simulink model "modelo_q1"  (R2016a)
settings: Solver=VariableStepAuto  StartTime=0.0  StopTime=20  MaxStep=0.001  RelTol=1e-3
values from neighbouring files (symbols this model uses):
  A = [(sin(th1)-sin(th1+2*th2))/(-3+cos(2*th2))  , (-sin(th1)+3*sin(th1+th2)-sin(th1-th2)+sin(th1+2*th2))/(-3+cos(2*th2)) ... (first row only)    [ajuda.m]    (also in controledesacoplante.m; gazebo_parameters.m = Amd; geracao.m = 0; gpc.m = [1.0013 0 0.0050)
  B = Bmd    [gazebo_parameters.m]    (also in geracao.m = 1; gpc.m = [-0.001; kalman_filter.m; questao1.m = double(subs(u, [x1 x2],[0 0])))
  C = Cm    [gazebo_parameters.m]    (also in geracao.m = -1; gpc.m = [1 0 0; kalman_filter.m; questao1.m = [1 0 0)
  D = 0    [geracao.m]    (also in gpc.m = zeros(3,1); questao1.m = zeros(3,1))
  Ka = lqr(A, B, Q, R)    [questao1.m]
  L = Lkf    [questao1.m]
  Lkf = dlqr(Amd',Cm',1e-4*eye(3),1*eye(2))'    [gazebo_parameters.m]    (also in kalman_filter.m; questao1.m = Lkf')
  V1 = 0.0001*eye(3)    [questao1.m]
  V2 = 0.000005*eye(2)    [questao1.m]
  x0 = [pi/180*30 0 0]    [questao1.m]
  x0obs = [pi/180*45 ; 0; 0]    [questao1.m]
undefined symbols (not defined in the file or in its folder): sigbuilder_block
libraries: simulink x5
settings Model: Creator=Regner  LastModifiedBy=Regner

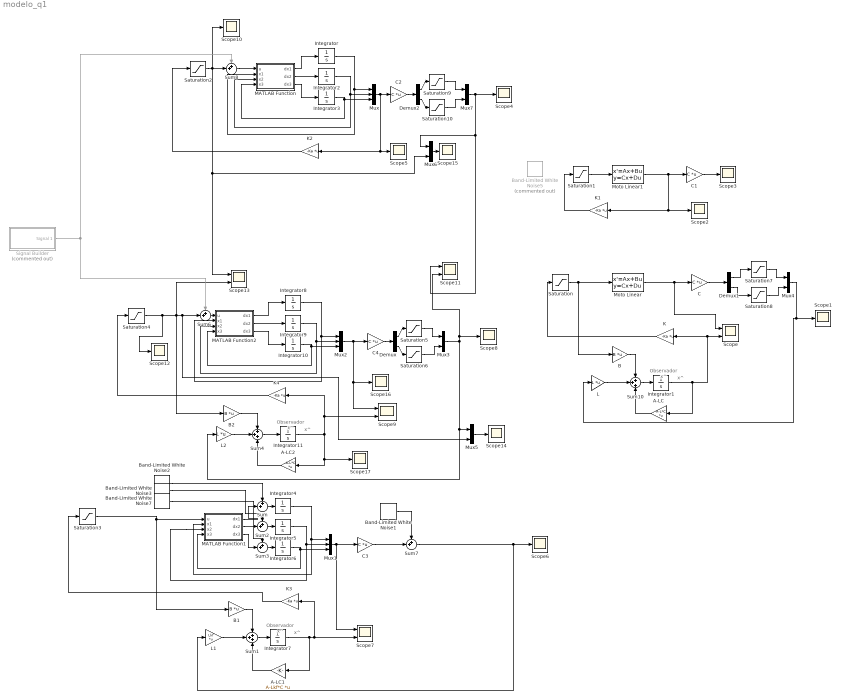
== system modelo_q1 ==
  note: Observador
  note: x^
  note: x^
  note: Observador
  note: x^
  note: x^
  note: Observador
  note: x^
  note: x^
  A-LC : Gain  Gain=A-L*C  Multiplication=Matrix(K*u)
  A-LC1 : Gain  Gain=A-Lkf*C  Multiplication=Matrix(K*u)
  A-LC2 : Gain  Gain=A-L*C  Multiplication=Matrix(K*u)
  B : Gain  Gain=B  Multiplication=Matrix(K*u)
  B1 : Gain  Gain=B  Multiplication=Matrix(K*u)
  B2 : Gain  Gain=B  Multiplication=Matrix(K*u)
  Band-Limited White Noise1 : simulink/Sources/Band-Limited White Noise  Cov=diag(V2)  Ts=0.1  seed=[23341]
  Band-Limited White Noise2 : simulink/Sources/Band-Limited White Noise  Cov=V1(1,1)  Ts=0.1  seed=[23341]
  Band-Limited White Noise3 : simulink/Sources/Band-Limited White Noise  Cov=V1(2,2)  Ts=0.1  seed=[23341]
  Band-Limited White Noise5 : simulink/Sources/Band-Limited White Noise  Commented=on  Cov=diag(V1)  Ts=0.1  seed=[23341]
  Band-Limited White Noise7 : simulink/Sources/Band-Limited White Noise  Cov=V1(3,3)  Ts=0.1  seed=[23341]
  C{,1..4} (5 alike) : Gain  Gain=C  Multiplication=Matrix(K*u)
  Demux : Demux  Outputs=2
  Demux1 : Demux  Outputs=2
  Demux2 : Demux  Outputs=2
  Integrator : Integrator  InitialCondition=x0(1)
  Integrator1 : Integrator  InitialCondition=x0obs
  Integrator10 : Integrator  InitialCondition=x0(3)
  Integrator11 : Integrator  InitialCondition=x0obs
  Integrator2 : Integrator  InitialCondition=x0(2)
  Integrator3 : Integrator  InitialCondition=x0(3)
  Integrator4 : Integrator  InitialCondition=x0(1)
  Integrator5 : Integrator  InitialCondition=x0(2)
  Integrator6 : Integrator  InitialCondition=x0(3)
  Integrator7 : Integrator  InitialCondition=x0obs
  Integrator8 : Integrator  InitialCondition=x0(1)
  Integrator9 : Integrator  InitialCondition=x0(2)
  K{,1..4} (5 alike) : Gain  Gain=-Ka  Multiplication=Matrix(K*u)
  L : Gain  Gain=L  Multiplication=Matrix(K*u)
  L1 : Gain  Gain=Lkf  Multiplication=Matrix(K*u)
  L2 : Gain  Gain=L  Multiplication=Matrix(K*u)
  MATLAB Function : MATLAB Function  TreatAsAtomicUnit=on
  MATLAB Function1 : MATLAB Function  TreatAsAtomicUnit=on
  MATLAB Function2 : MATLAB Function  TreatAsAtomicUnit=on
  Moto Linear : StateSpace  A=A  B=B  C=eye(3)  D=D  X0=x0
  Moto Linear1 : StateSpace  A=A  B=B  C=eye(3)  D=D  X0=x0
  Mux : Mux  Inputs=3
  Mux1 : Mux  Inputs=3
  Mux2 : Mux  Inputs=3
  Mux{3..7} (5 alike) : Mux  Inputs=2
  Saturation : Saturate  UpperLimit=50  LowerLimit=-50  ZeroCross=off
  Saturation1 : Saturate  UpperLimit=100  LowerLimit=-100  ZeroCross=off
  Saturation{5..6,9..10} (4 alike) : Saturate  UpperLimit=pi/4  LowerLimit=-pi/4
  Saturation2 : Saturate  UpperLimit=pi/2  LowerLimit=-pi/2  ZeroCross=off
  Saturation3 : Saturate  UpperLimit=inf  LowerLimit=-inf  ZeroCross=off
  Saturation4 : Saturate  UpperLimit=100  LowerLimit=-100  ZeroCross=off
  Saturation7 : Saturate  UpperLimit=pi  LowerLimit=-pi
  Saturation8 : Saturate  UpperLimit=pi  LowerLimit=-pi
  Scope{,7,9,11,13} (5 alike) : Scope  NumInputPorts=2
  Scope{1..6,8,10,12,14..17} (13 alike) : Scope
  Signal Builder : Subsystem  Tag=STV Subsys  Commented=on  LoadFcn=sigbuilder_block('load');  StartFcn=sigbuilder_block('start');  StopFcn=sigbuilder_block('stop');  ClipboardFcn=sigbuilder_block('clipboard');  mask(Sigbuilder block){}
      mask help: Simulink:masks:SigbuilderBlock_MD
      mask init:
      | if ~strcmp(get_param(bdroot(gcbh),'SimulationStatus'),'stopped') tuvar = sigbuilder_block('maskInit'); end
      settings: CopyFcn=sigbuilder_block('copy');  DeleteFcn=sigbuilder_block('delete');  ModelCloseFcn=sigbuilder_block('modelClose');  PreSaveFcn=sigbuilder_block('preSave');  PauseFcn=sigbuilder_block('pause');  ContinueFcn=sigbuilder_block('continue');  NameChangeFcn=sigbuilder_block('namechange');  OpenFcn=sigbuilder_block('open',[437.6 199.2 550.4 400 ]);  CloseFcn=sigbuilder_block('close');
      mask Display: plot(0, 0, 100, 100,[2, 2, 32, 32, 2], [68, 8, 8, 68, 68],[32, 2], [38, 38], [32, 19, 2],[53, 60, 44], [32, 17, 17, 2],[16, 16, 31, 31]);txt = getActiveGroup(gcbh);text(2, 100, txt,'verticalAlignment', 'top');
  Sum{,2..3,6..8} (6 alike) : Sum  Inputs=++|
  Sum1 : Sum  Inputs=+++
  Sum10 : Sum  Inputs=+++
  Sum4 : Sum  Inputs=+++
  wires:
  Moto Linear/1 -> C/1, Scope/1
  K/1 -> Saturation/1
  Mux4/1 -> L/1, Scope1/1
  Saturation1/1 -> Moto Linear1/1
  Moto Linear1/1 -> C1/1, Scope2/1, K1/1
  K1/1 -> Saturation1/1
  C1/1 -> Scope3/1
  Sum10/1 -> Integrator1/1
  L/1 -> Sum10/2
  A-LC/1 -> Sum10/3
  Integrator1/1 -> A-LC/1, Scope/2, K/1
  B/1 -> Sum10/1
  MATLAB Function/1(dx1) -> Integrator/1
  MATLAB Function/2(dx2) -> Integrator2/1
  MATLAB Function/3(dx3) -> Integrator3/1
  Integrator3/1 -> Mux/3, MATLAB Function/4(x3)
  Integrator2/1 -> Mux/2, MATLAB Function/3(x2)
  Integrator/1 -> Mux/1, MATLAB Function/2(x1)
  Saturation2/1 -> Sum8/2, Mux6/2, Scope13/1, Scope10/1
  Mux/1 -> Scope5/1, K2/1, C2/1
  K2/1 -> Saturation2/1
  MATLAB Function1/1(dx1) -> Sum/2
  MATLAB Function1/2(dx2) -> Sum2/2
  MATLAB Function1/3(dx3) -> Sum3/2
  K3/1 -> Saturation3/1
  Sum7/1 -> L1/1, Scope6/1
  Mux1/1 -> Scope7/1, C3/1
  Sum1/1 -> Integrator7/1
  L1/1 -> Sum1/2
  A-LC1/1 -> Sum1/3
  Integrator7/1 -> K3/1, Scope7/2, A-LC1/1
  B1/1 -> Sum1/1
  Band-Limited White Noise1/1 -> Sum7/1
  Saturation3/1 -> MATLAB Function1/1(u), B1/1
  MATLAB Function2/1(dx1) -> Integrator8/1
  MATLAB Function2/2(dx2) -> Integrator9/1
  MATLAB Function2/3(dx3) -> Integrator10/1
  Integrator10/1 -> Mux2/3, MATLAB Function2/4(x3)
  Integrator9/1 -> Mux2/2, MATLAB Function2/3(x2)
  Integrator8/1 -> Mux2/1, MATLAB Function2/2(x1)
  K4/1 -> Saturation4/1
  Mux3/1 -> Mux5/1, L2/1, Scope11/2, Scope8/1
  Saturation4/1 -> Scope12/1, Mux5/2, Sum6/2, Scope13/2, B2/1
  Mux2/1 -> C4/1, Scope16/1, Scope9/1
  Sum4/1 -> Integrator11/1
  L2/1 -> Sum4/2
  A-LC2/1 -> Sum4/3
  Integrator11/1 -> K4/1, Scope9/2, Scope17/1, A-LC2/1
  B2/1 -> Sum4/1
  Saturation/1 -> B/1, Moto Linear/1
  Integrator4/1 -> MATLAB Function1/2(x1), Mux1/1
  Integrator5/1 -> MATLAB Function1/3(x2), Mux1/2
  Integrator6/1 -> MATLAB Function1/4(x3), Mux1/3
  Band-Limited White Noise7/1 -> Sum3/1
  Band-Limited White Noise3/1 -> Sum2/1
  Band-Limited White Noise2/1 -> Sum/1
  C3/1 -> Sum7/2
  Mux7/1 -> Scope11/1, Mux6/1, Scope4/1
  Sum6/1 -> MATLAB Function2/1(u)
  Sum8/1 -> MATLAB Function/1(u)
  Signal Builder/1(Signal 1) -> Sum6/1, Sum8/1
  C4/1 -> Demux/1
  Demux/1 -> Saturation5/1
  Demux/2 -> Saturation6/1
  Saturation6/1 -> Mux3/2
  Saturation5/1 -> Mux3/1
  C/1 -> Demux1/1
  Demux1/1 -> Saturation7/1
  Demux1/2 -> Saturation8/1
  Saturation8/1 -> Mux4/2
  Saturation7/1 -> Mux4/1
  Mux5/1 -> Scope14/1
  Mux6/1 -> Scope15/1
  C2/1 -> Demux2/1
  Demux2/1 -> Saturation9/1
  Demux2/2 -> Saturation10/1
  Saturation10/1 -> Mux7/2
  Saturation9/1 -> Mux7/1
  Sum/1 -> Integrator4/1
  Sum2/1 -> Integrator5/1
  Sum3/1 -> Integrator6/1

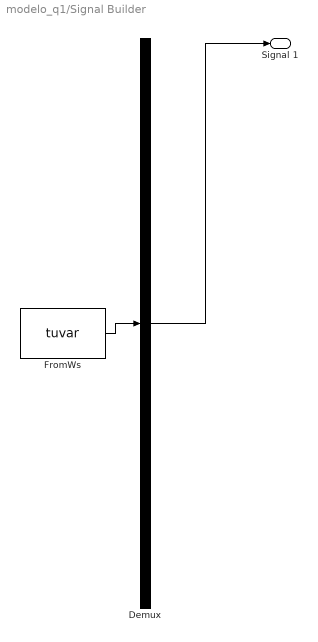
== system modelo_q1/Signal Builder ==
  Demux : Demux  Tag=STV Demux  Outputs=1
  FromWs : FromWorkspace  Tag=STV FromWs  VariableName=tuvar  SampleTime=0
      SigBuilderData=|
      | common.afterFinalStr = 'Extrapolate'
      | common.sampleTime = 0
      | dataSet.timeRange = [0 20]
      | dataSet.name = 'Group 1'
      | sbobj.Groups.Name = 'Group 1'
      | sbobj.Groups.Signals.Name = 'Signal 1'
      | sbobj.Groups.Signals.XData = [0 4 4 4.5 4.5 10 10 12 12 17.5 17.5 18 18 20]
      | sbobj.Groups.Signals.YData = [0 0 0.2 0.2 0 0 0.12 0.12 0 0 0.474 0.474 0 0]
      | sbobj.Groups.TimeRange = [0 20]
  Signal 1 : Outport  Tag=STV Outport
  wires:
  Demux/1 -> Signal 1/1
  FromWs/1 -> Demux/1

== matlab function modelo_q1/MATLAB Function1 ==
  data: u input; dx1 output; x1 input; x2 input; x3 input; dx2 output; dx3 output
function [dx1,dx2,dx3] = fcn(u, x1, x2, x3)
% Parâmetros do modelo
Mv = 0.152; % Massa do veículo sem giro [kg]
Mg = 0.15; % Massa do giro [kg]
Rg = 0.095/2; % Raio do giro [m]
Ag = 0.006; % Espessura giro [m]
Av = 0.075; % Altura veículo [m]
Lv = 0.19; % Largura veículo [m]
Dg = 0.06; % Distância entre centro de massa do giro e eixo de rotação [m]
Dv = 0.045; % Distância entre centro de massa do veículo e eixo de rotação
Omega = 7200*0.10472; % Velocidade de rotação do giro, rpm*conversão = rad/sec
g = 9.81; % Gravidade [m/s^2] 
IG11 = Mg*(Rg^2)/4 + Mg*(Ag^2)/12; % Algum momento de inercia
IG33 = Mg*(Rg^2)/2;
IB11 = Mv*(Av^2+Lv^2)/12;

dx1 = x3;
dx2 = 0 + u;
dx3 = ((Mv*Dv+Mg*Dg)*g*sin(x1))/(IB11+Mv*(Dv^2)+IG11*(cos(x2)^2)+Mg*(Dg^2)+IG33*((sin(x2))^2))+u*(-2*cos(x2)*sin(x2)*x3*(IG33-IG11)-Omega*cos(x2)*IG33)/(IB11+IG11*(cos(x2)^2)+Mv*(Dv^2)+Mg*(Dg^2)+IG33*(sin(x2)^2));

== matlab function modelo_q1/MATLAB Function ==
  data: u input; dx1 output; x1 input; x2 input; x3 input; dx2 output; dx3 output
function [dx1,dx2,dx3] = fcn(u, x1, x2, x3)
% Parâmetros do modelo
Mv = 0.152; % Massa do veículo sem giro [kg]
Mg = 0.15; % Massa do giro [kg]
Rg = 0.095/2; % Raio do giro [m]
Ag = 0.006; % Espessura giro [m]
Av = 0.075; % Altura veículo [m]
Lv = 0.19; % Largura veículo [m]
Dg = 0.06; % Distância entre centro de massa do giro e eixo de rotação [m]
Dv = 0.045; % Distância entre centro de massa do veículo e eixo de rotação
Omega = 7200*0.10472; % Velocidade de rotação do giro, rpm*conversão = rad/sec
g = 9.81; % Gravidade [m/s^2] 
IG11 = Mg*(Rg^2)/4 + Mg*(Ag^2)/12; % Algum momento de inercia
IG33 = Mg*(Rg^2)/2;
IB11 = Mv*(Av^2+Lv^2)/12;

dx1 = x3;
dx2 = 0 + u;
dx3 = ((Mv*Dv+Mg*Dg)*g*sin(x1))/(IB11+Mv*(Dv^2)+IG11*(cos(x2)^2)+Mg*(Dg^2)+IG33*((sin(x2))^2))+u*(-2*cos(x2)*sin(x2)*x3*(IG33-IG11)-Omega*cos(x2)*IG33)/(IB11+IG11*(cos(x2)^2)+Mv*(Dv^2)+Mg*(Dg^2)+IG33*(sin(x2)^2));

== matlab function modelo_q1/MATLAB Function2 ==
  data: u input; dx1 output; x1 input; x2 input; x3 input; dx2 output; dx3 output
function [dx1,dx2,dx3] = fcn(u, x1, x2, x3)
% Parâmetros do modelo
Mv = 0.152; % Massa do veículo sem giro [kg]
Mg = 0.15; % Massa do giro [kg]
Rg = 0.095/2; % Raio do giro [m]
Ag = 0.006; % Espessura giro [m]
Av = 0.075; % Altura veículo [m]
Lv = 0.19; % Largura veículo [m]
Dg = 0.06; % Distância entre centro de massa do giro e eixo de rotação [m]
Dv = 0.045; % Distância entre centro de massa do veículo e eixo de rotação
Omega = 7200*0.10472; % Velocidade de rotação do giro, rpm*conversão = rad/sec
g = 9.81; % Gravidade [m/s^2] 
IG11 = Mg*(Rg^2)/4 + Mg*(Ag^2)/12; % Algum momento de inercia
IG33 = Mg*(Rg^2)/2;
IB11 = Mv*(Av^2+Lv^2)/12;

dx1 = x3;
dx2 = 0 + u;
dx3 = ((Mv*Dv+Mg*Dg)*g*sin(x1))/(IB11+Mv*(Dv^2)+IG11*(cos(x2)^2)+Mg*(Dg^2)+IG33*((sin(x2))^2))+u*(-2*cos(x2)*sin(x2)*x3*(IG33-IG11)-Omega*cos(x2)*IG33)/(IB11+IG11*(cos(x2)^2)+Mv*(Dv^2)+Mg*(Dg^2)+IG33*(sin(x2)^2));
